simulink model "lews_model_static_backup"  (R2026a)
settings: Solver=VariableStepAuto  StopTime=7200
values from neighbouring files (symbols this model uses):
  beta_deg = varargin{1}    [lews_physics.m]    (also in main.m = 42)
  c_prime = p.c_prime    [lews_physics.m]    (also in main.m = 7; plot_results.m = 12)
settings Model: Creator=HARIKRISHNAN  LastModifiedBy=HARIKRISHNAN

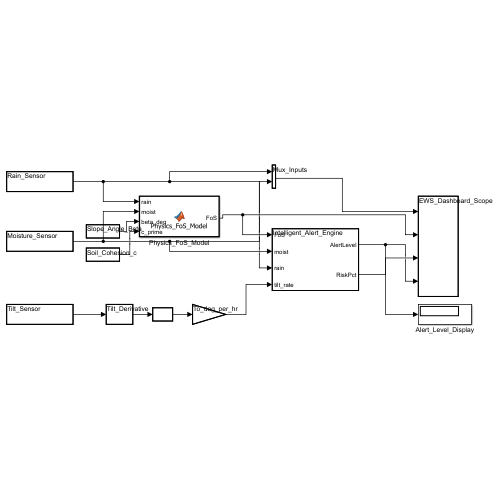
[thumbnail: Simulink's stored preview of the top-level diagram]
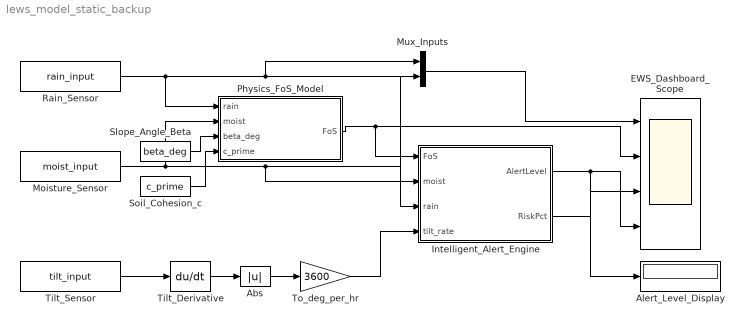
== system lews_model_static_backup ==
  Abs : Abs  SaturateOnIntegerOverflow=off
  Alert_Level_Display : Display
  EWS_Dashboard_Scope : Scope  NumInputPorts=4
      settings: ActiveDisplayString=4  Title=4. Alert Level (0=Safe, 1=Advisory, 2=Evacuate)  ActiveDisplayYMinimum=-0.2  ActiveDisplayYMaximum=2.2
  Intelligent_Alert_Engine : MATLAB Function  TreatAsAtomicUnit=on
  Moisture_Sensor : FromWorkspace  VariableName=moist_input
  Mux_Inputs : Mux  Inputs=2
  Physics_FoS_Model : MATLAB Function  TreatAsAtomicUnit=on
  Rain_Sensor : FromWorkspace  VariableName=rain_input
  Slope_Angle_Beta : Constant  Value=beta_deg
  Soil_Cohesion_c : Constant  Value=c_prime
  Tilt_Derivative : Derivative
  Tilt_Sensor : FromWorkspace  VariableName=tilt_input
  To_deg_per_hr : Gain  Gain=3600
  wires:
  Rain_Sensor/1 -> Intelligent_Alert_Engine/3(rain), Mux_Inputs/1, Physics_FoS_Model/1(rain)
  Moisture_Sensor/1 -> Intelligent_Alert_Engine/2(moist), Mux_Inputs/2, Physics_FoS_Model/2(moist)
  Tilt_Sensor/1 -> Tilt_Derivative/1
  Tilt_Derivative/1 -> Abs/1
  Abs/1 -> To_deg_per_hr/1
  Physics_FoS_Model/1(FoS) -> Intelligent_Alert_Engine/1(FoS), EWS_Dashboard_Scope/2
  To_deg_per_hr/1 -> Intelligent_Alert_Engine/4(tilt_rate)
  Mux_Inputs/1 -> EWS_Dashboard_Scope/1
  Intelligent_Alert_Engine/2(RiskPct) -> EWS_Dashboard_Scope/3
  Intelligent_Alert_Engine/1(AlertLevel) -> EWS_Dashboard_Scope/4, Alert_Level_Display/1
  Slope_Angle_Beta/1 -> Physics_FoS_Model/3(beta_deg)
  Soil_Cohesion_c/1 -> Physics_FoS_Model/4(c_prime)

== matlab function lews_model_static_backup/Intelligent_Alert_Engine ==
  data: FoS input; AlertLevel output; moist input; rain input; tilt_rate input; RiskPct output
function [AlertLevel, RiskPct] = Intelligent_Alert_Engine(FoS, moist, rain, tilt_rate)
% Persistent variable to handle alert state and avoid flickering
persistent current_state;
if isempty(current_state)
    current_state = 0;
end

% Continuous Risk Percentage calculation (0 to 100%)
fos_risk = max(0, min(100, (1.8 - FoS) * 100));
kinematic_risk = min(100, tilt_rate * 20);
moist_risk = max(0, (moist - 0.25) * 250);
RiskPct = max(0, min(100, 0.4*fos_risk + 0.35*kinematic_risk + 0.25*moist_risk));

% Multi-tier Warning Levels with Hysteresis:
% 0 = Green (Safe), 1 = Yellow (Advisory), 2 = Red (Evacuate)
if current_state == 0
    if RiskPct >= 50 || FoS < 1.15 || tilt_rate > 3.0
        current_state = 1;
    end
elseif current_state == 1
    if RiskPct >= 80 || FoS < 1.0 || (FoS < 1.1 && tilt_rate > 2.0)
        current_state = 2;
    elseif RiskPct < 35 && FoS > 1.3 && tilt_rate < 1.0
        current_state = 0;
    end
elseif current_state == 2
    if RiskPct < 60 && FoS > 1.25
        current_state = 1;
    end
end
AlertLevel = current_state;
end

== matlab function lews_model_static_backup/Physics_FoS_Model ==
  data: rain input; FoS output; moist input; beta_deg input; c_prime input
function FoS = Physics_FoS_Model(rain, moist, beta_deg, c_prime)
% Slope and Geotechnical Constants
phi_rad = deg2rad(30);
beta_rad = deg2rad(beta_deg);
gamma_s = 18;     % kN/m^3
gamma_w = 9.81;   % kN/m^3
z = 1.5;          % meters

% Pore pressure estimation
theta_crit = 0.35;
if moist > theta_crit
    u = gamma_w * (moist - theta_crit) * z * 2.5 + (rain * 0.02);
else
    u = 0;
end

normal_stress = gamma_s * z * (cos(beta_rad))^2;
eff_stress = max(normal_stress - u, 0.1);
resisting_shear = c_prime + eff_stress * tan(phi_rad);
driving_shear = gamma_s * z * sin(beta_rad) * cos(beta_rad);
FoS = resisting_shear / max(driving_shear, 0.001);
end
